simulink model "multirate_d4_cauer2_pc"  (Simulink 4.00)
settings: Solver=FixedStepDiscrete  SolverMode=SingleTasking  StartTime=0.0  StopTime=5.0  RelTol=1e-3
undefined symbols (not defined in the file or in its folder): a, b
libraries: dspbuff3 x2, dspsigops x2, dspsrcs3 x1, dspsnks3 x1
settings Model: LastModifiedBy=wir  LimitDataPoints=off  RTWSystemTargetFile=ert.tlc  RTWTemplateMakefile=ert_default_tmf  RTWGenerateCodeOnly=on  ExtModeMexFile=no_ext_comm

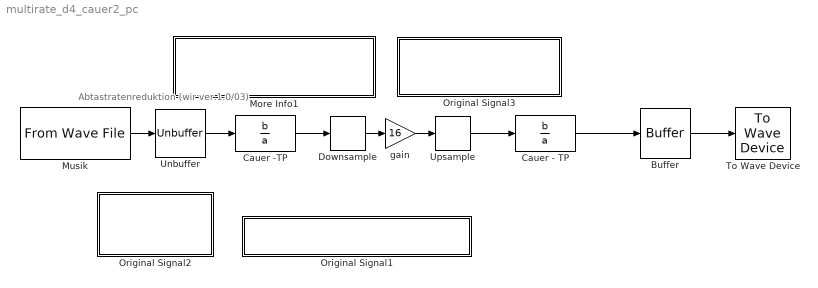
== system multirate_d4_cauer2_pc ==
  note: Abtastratenreduktion
      | (wir ver.1.0/03)
  " Cauer - TP " : DiscreteFilter  Numerator=b  Denominator=a  SampleTime=-1  Realization=auto
      settings: RTWStateStorageClass=Auto
  " Cauer -TP " : DiscreteFilter  Numerator=b  Denominator=a  SampleTime=-1  Realization=auto
      settings: RTWStateStorageClass=Auto
  Buffer : dspbuff3/Buffer  N=256  V=0  ic=0
  Downsample : dspsigops/Downsample  N=4  phase=0  ic=0  smode=Allow multirate  fmode=Maintain input frame size
  More Info1 : Subsystem
      settings: RTWFcnNameOpts=Auto  RTWFileNameOpts=Auto
      mask Display: disp(' Aufgaben')
  Musik : dspsrcs3/From Wave File  FileName=speech_dft  SamplesPerFrame=256  MinBufSize=256
  Original Signal1 : Subsystem  Description=Filterentwurf übernehmen
      settings: OpenFcn=[b,a] = filtdemo('getfilt')  RTWFcnNameOpts=Auto  RTWFileNameOpts=Auto
      mask Type: Cauer-Filter
      mask Display: disp('Momentanen Entwurf übernehmen')
  Original Signal2 : Subsystem  Description=Filterentwurf
      settings: OpenFcn=filtdemo  RTWFcnNameOpts=Auto  RTWFileNameOpts=Auto
      mask Type: Cauer-Filter
      mask Display: disp('Filterentwurf')
  Original Signal3 : Subsystem  Description=Initialisierung Cauer-Filter
      settings: OpenFcn="b = [    0.0237    0.0129    0.0129    0.0237] ; a = [  1.0000   -2.2668    2.0908   -0.7508];"  RTWFcnNameOpts=Auto  RTWFileNameOpts=Auto
      mask Type: Cauer-Filter
      mask Display: disp('Init default Cauer-Filter')
  To Wave Device : dspsnks3/To Wave Device  bufDuration=2  initDelay=0.1  useDefaultDevice=on  userDeviceID=1
  Unbuffer : dspbuff3/Unbuffer  ic=0
  Upsample : dspsigops/Upsample  N=4  phase=0  ic=0  mode=Maintain input frame size
  gain : Gain  Gain=16  Multiplication=Element-wise(K.*u)  SaturateOnIntegerOverflow=on
  wires:
  ? -> ?
  gain/1 -> Upsample/1
  " Cauer - TP "/1 -> Buffer/1
  " Cauer -TP "/1 -> Downsample/1
  Musik/1 -> Unbuffer/1
  Unbuffer/1 -> " Cauer -TP "/1
  Downsample/1 -> gain/1
  Upsample/1 -> " Cauer - TP "/1
  Buffer/1 -> To Wave Device/1

== system multirate_d4_cauer2_pc/More Info1 ==
  note: Abtastratenreduktion
      | (B.Wir 23.5.03 ver  0.1)
      |
      | Cauer-Filter sind für die Audioverarbeitung besonders geeignet, da sie eine hohe
      | Flankensteilheit bei geringer Filterordnung ermöglichen.
      | Die nichtlineare Phase der Cauer-Filter ist wegen dee Phasentaubheit des Gehörs unwesentlich.
      |
      | Mit den Feld 'Filterentwurf' können Sie unterschiedliche Filterentwurfmethoden testen.
      | Die Übernahme der Filterkoeffizienten erfolgt bei geöffneten Entwurfsfenster!
      |
      |
      | Aufgaben:
      |
      | 0) Doppelklick auf das Feld 'Default Cauer-Filter' initialisiert die beiden grünen  Cauer-Tiefpässe.
      |     Starten Sie die Simulation!
      |     Starten Sie den Filterentwurf. Welche Grenzfrequenz und welche Sperrdämfung sind sinnvoll?
      |     Schätzen Sie den Rechenzeitbedarf bei einem  Elliptischen (Cauer-), Fenster- und REMEZ-Entwurf ab!
      |
      | 1) Entfernen Sie den grünen Cauer-Tiefpass am Ausgang und starten Sie die Simulation. Erklären Sie
      |     die Störungen indem Sie den Betrag des Signalspektrumdurch entlang der Signalkette skizzieren.
      |
      | 2) Entfernen Sie nun zusätzlich den  Cauer-Tiefpass am Eingang und erklären Sie die Störungen.
      |
      | 3) Entfernen Sie nur den  Cauer-Tiefpass am Eingang und erklären Sie die Störungen.

== system multirate_d4_cauer2_pc/Original Signal1 ==

== system multirate_d4_cauer2_pc/Original Signal2 ==

== system multirate_d4_cauer2_pc/Original Signal3 ==
